simulink model "dspddc"  (Simulink 6.0)
settings: Solver=FixedStepDiscrete  SolverMode=SingleTasking  StartTime=0.0  StopTime=20500/69.333e6  RelTol=1e-3
PreLoadFcn:
  | gsmcoeffs
InitFcn:
  | ;fxptdlg('fxptdlg_simInit_cb');
StartFcn:
  | ;fxptdlg('fxptdlg_sim_cb');
StopFcn:
  | ;fxptdlg('fxptdlg_store_cb');
values from neighbouring files (symbols this model uses):
  cfir = [ -0.00073242187500  -0.00091552734375   0.00393676757813            0.01202392578125   0.00631713867188  -0.02673339843750           -0.05920410156250  -0.02371215820313   0.11474609375000            0.28945922851563   0.37011718750000   0.28945922851563            0.11474609375000  -0.02371215820313  -0.05920410156250           -0.02673339843750   0.00631713867188   0.01202392578125            0 ...(+54 chars)    [gsmcoeffs.m]
  pfir = [0.00073242187500   0.00213623046875  -0.00024414062500    -0.00253295898438  -0.00265502929688   0.00125122070313     0.00494384765625   0.00320434570313  -0.00338745117188     -0.00744628906250  -0.00314331054688   0.00601196289063    0.00991821289063   0.00292968750000  -0.00885009765625    -0.01293945312500  -0.00320434570313   0.01242065429688    0.01766967773438   0.00396728515625  -0.018188 ...(+835 chars)    [gsmcoeffs.m]
libraries: simulink x9, dspmlti3 x4, dspsigops x3, dspbuff3 x1, dspmlti4 x1, fixpt_lib_4 x1, dspsrcs4 x1, dspsnks4 x1, dspindex x1
PreSaveFcn:
  | ;fxptdlg('fxptdlg_presave_cb');
CloseFcn:
  | ;fxptdlg('fxptdlg_close_cb');
settings Model: MinMaxOverflowLogging=OverflowOnly  Creator=schim  LastModifiedBy=sconahan  ExtModeAutoUpdateStatusClock=off  ProdHWDeviceType=ASIC/FPGA
settings DataIOCC: LimitDataPoints=off  SaveOutput=off  SaveTime=off  SignalLoggingName=sigsOut
settings OptimizationCC: InlineParams=on
settings DebuggingCC: CheckExecutionContextPreStartOutputMsg=on  CheckExecutionContextRuntimeOutputMsg=on  SolverPrmCheckMsg=none  IntegerOverflowMsg=none  ParameterPrecisionLossMsg=none
settings HardwareCC: ProdHWDeviceType=ASIC/FPGA

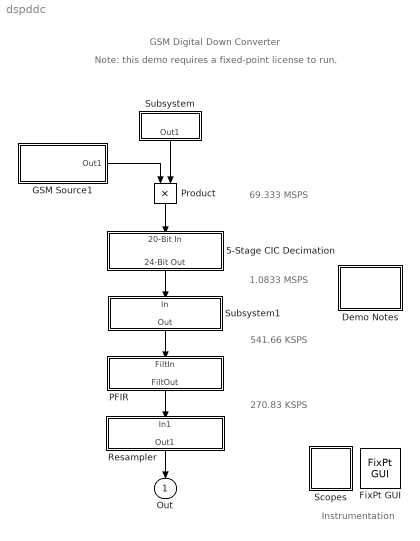
== system dspddc ==
  note: 1.0833
      | MSPS
  note: 541.66
      | KSPS
  note: 270.83
      | KSPS
  note: 69.333
      | MSPS
  note: Instrumentation
  note: GSM Digital Down Converter
  note: Note: this demo requires a fixed-point license to run.
  5-Stage CIC Decimation : Subsystem  Orientation=down  PropExecContextAcrossSSBoundary=on
      mask Display: disp('CIC Decimator')
  Demo Notes : Subsystem  PropExecContextAcrossSSBoundary=on
      settings: OpenFcn=web(which('dspddc.html'))
      mask Display: disp('Notes')
  FixPt GUI : fixpt_lib_4/FixPt GUI
  GSM Source1 : Subsystem  PropExecContextAcrossSSBoundary=on  mask(GSM Source){source_type=Chirp}
      mask prompts: source_type "Source type:"
      mask init:
      | pure_tune_input = (source_type - 1);
      mask StyleString: popup(Chirp|Sinusoid)
      mask Display:
      | disp(['GSM' 10 'Source']);
      | 
      | 
      | 
      | 
      | 
      | 
      | port_label('output', 1, 'A/D');
  PFIR : Subsystem  Orientation=down  PropExecContextAcrossSSBoundary=on  mask(PFIR){h=pfir, g=1024}
      mask prompts: h "PFIR coefficients:"; g "FINE gain (1-16383):"
      mask help: Valid FINE (gain parameter) inputs are positive integers less than 16383. The FINE_GAIN is calculated as FINE/1024.
      mask Display: disp('Programmable FIR')
  Product : Product  Orientation=down  OutDataTypeMode=Specify via dialog  OutDataType=sfix(20)  OutScaling=2^-18  RndMeth=Nearest
  Resampler : Subsystem  Orientation=down  PropExecContextAcrossSSBoundary=on  mask(Resampler){h=fir1(31,0.25), Ndelay=4, Ndec=3}
      mask prompts: h "Resampling FIR coefficients:"; Ndelay "NDELAY (upsample factor):"; Ndec "NDEC (downsample factor):"
      mask Display: disp('Rate Conversion')
  Scopes : Subsystem  PropExecContextAcrossSSBoundary=on
      mask Display: disp('Scopes')
  Subsystem : Subsystem  Orientation=down  PropExecContextAcrossSSBoundary=on  mask(Numerically Controlled Oscillator (NCO)){tune_freq=(5/24) * (2^32), phase_offset=0, enable_dither=on, bits=5}
      mask prompts: tune_freq "Normalized 32-bit tuning frequency (0 to 2^32)"; phase_offset "Normalized 16-bit phase offset (0 to 2^16):"; enable_dither "Enable dithering"; bits "Number of dither bits (1 to 19):"
      mask Display: disp('NCO')
  Subsystem1 : Subsystem  Orientation=down  PropExecContextAcrossSSBoundary=on  mask(Compensation FIR (CFIR)){coarse_gain=0, cfir_h=cfir}
      mask prompts: coarse_gain "COARSE gain (0-7):"; cfir_h "CFIR coefficients:"
      mask Display: disp('Compensation FIR')
  Out : Outport  Orientation=down
  wires:
  Product/1 -> 5-Stage CIC Decimation/1(20-Bit In)
  Subsystem/1(Out1) -> Product/2
  GSM Source1/1(Out1) -> Product/1
  Subsystem1/1(Out) -> PFIR/1(FiltIn)
  PFIR/1(FiltOut) -> Resampler/1(In1)
  Resampler/1(Out1) -> Out/1
  5-Stage CIC Decimation/1(24-Bit Out) -> Subsystem1/1(In)

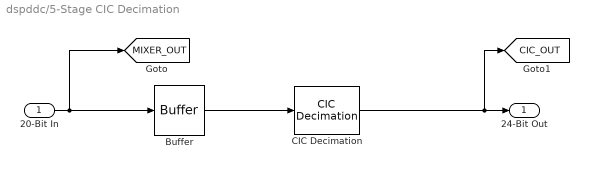
== system dspddc/5-Stage CIC Decimation ==
  20-Bit In : Inport  LatchInput=off
  Buffer : dspbuff3/Buffer  N=64  V=0  ic=0
  CIC Decimation : dspmlti4/CIC Decimation  filtFrom=Dialog  filtobj=Hm_decim  ftype=Decimator  R=64  resampPhase=0  M=1  N=5  BPS=[50 29 24 24 24 24 24 24 24 24]  launchFVT=off  framing=Maintain input frame rate
  24-Bit Out : Outport
  tag scope: CIC_OUT=global, MIXER_OUT=global
  wires:
  20-Bit In/1 -> [MIXER_OUT], Buffer/1
  Buffer/1 -> CIC Decimation/1
  CIC Decimation/1 -> 24-Bit Out/1, [CIC_OUT]

== system dspddc/Demo Notes ==

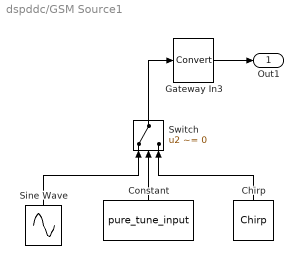
== system dspddc/GSM Source1 ==
  Chirp : dspsrcs4/Chirp  Orientation=up  sweep=Linear  mode=Unidirectional  f0=.2078*69.333e6  f1=.2088*69.333e6  t1=16384/69.333e6  Tsweep=16384/69.333e6  phase=0  Ts=1/69.333e6  spf=1  datatype=Double
  Constant : Constant  Orientation=up  Value=pure_tune_input  OutDataTypeMode=boolean
  Gateway In3 : DataTypeConversion  OutDataTypeMode=Specify via dialog  OutDataType=sfix(14)  OutScaling=2^-13  RndMeth=Nearest  SaturateOnIntegerOverflow=on
  Sine Wave : Sin  Orientation=up  Frequency=2*pi*69.1e6*5/24  SampleTime=1/69.333e6
  Switch : Switch  Orientation=up  Criteria=u2 ~= 0  Threshold=0.5  InputSameDT=on
  Out1 : Outport
  wires:
  Switch/1 -> Gateway In3/1
  Sine Wave/1 -> Switch/1
  Chirp/1 -> Switch/3
  Constant/1 -> Switch/2
  Gateway In3/1 -> Out1/1

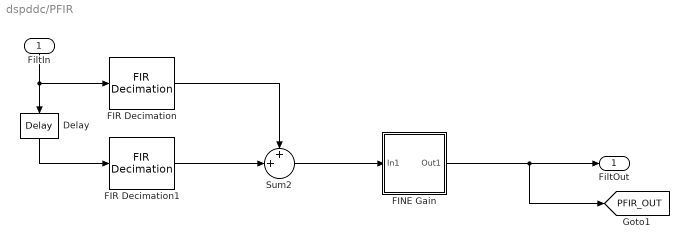
== system dspddc/PFIR ==
  FiltIn : Inport  Orientation=down  LatchInput=off
  Delay : dspsigops/Delay  Orientation=down  dly_unit=Samples  delay=1  ic_detail=off  dif_ic_for_ch=off  dif_ic_for_dly=off  ic=0  reset_popup=None
  FINE Gain : Subsystem  PropExecContextAcrossSSBoundary=on
      mask Display: disp('FINE\nGain')
  FIR Decimation : dspmlti3/FIR Decimation  DialogController=dspDDGCreate  DialogControllerArgs=DataTag1  h=h(1:2:length(h))  D=2  framing=Maintain input frame size  outputBufInitCond=0  firstCoeffMode=Specify word length  firstCoeffWordLength=16  firstCoeffFracLength=16  prodOutputMode=Binary point scaling  prodOutputWordLength=20  prodOutputFracLength=-12  roundingMode=Nearest  overflowMode=off
  FIR Decimation1 : dspmlti3/FIR Decimation  DialogController=dspDDGCreate  DialogControllerArgs=DataTag2  h=h(2:2:length(h))  D=2  framing=Maintain input frame size  outputBufInitCond=0  firstCoeffMode=Specify word length  firstCoeffWordLength=16  firstCoeffFracLength=16  prodOutputMode=Binary point scaling  prodOutputWordLength=20  prodOutputFracLength=-12  roundingMode=Nearest  overflowMode=off
  Sum2 : Sum  Inputs=++|  OutDataType=sfix(20)  OutScaling=2^12  SaturateOnIntegerOverflow=on  InputSameDT=on
  FiltOut : Outport
  tag scope: PFIR_OUT=global
  wires:
  Delay/1 -> FIR Decimation1/1
  FIR Decimation/1 -> Sum2/1
  FIR Decimation1/1 -> Sum2/2
  FiltIn/1 -> Delay/1, FIR Decimation/1
  Sum2/1 -> FINE Gain/1(In1)
  FINE Gain/1(Out1) -> FiltOut/1, [PFIR_OUT]

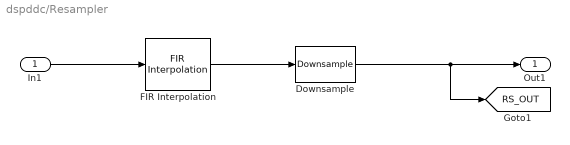
== system dspddc/Resampler ==
  In1 : Inport  LatchInput=off
  Downsample : dspsigops/Downsample  N=Ndec  phase=0  ic=0  smode=Allow multirate  fmode=Maintain input frame size
  FIR Interpolation : dspmlti3/FIR Interpolation  DialogController=dspDDGCreate  DialogControllerArgs=DataTag3  h=h  L=Ndelay  framing=Maintain input frame size  outputBufInitCond=0  firstCoeffMode=Specify word length  firstCoeffWordLength=12  firstCoeffFracLength=13  prodOutputMode=Binary point scaling  prodOutputWordLength=24  prodOutputFracLength=-12  roundingMode=Nearest  overflowMode=off
  Out1 : Outport
  tag scope: RS_OUT=global
  wires:
  In1/1 -> FIR Interpolation/1
  Downsample/1 -> [RS_OUT], Out1/1
  FIR Interpolation/1 -> Downsample/1

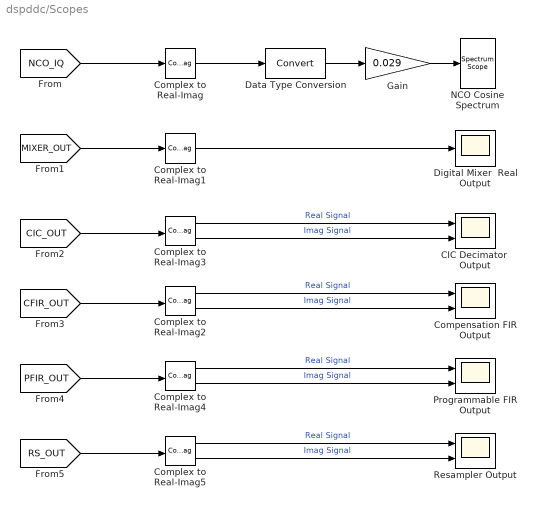
== system dspddc/Scopes ==
  CIC Decimator  Output : Scope  NumInputPorts=2
      settings: TimeRange=0.0003  YMin=-1e+009~-1e+009  YMax=1e+009~1e+009  DataFormat=Structure  MaxDataPoints=1000000
  Compensation FIR Output : Scope  NumInputPorts=2
      settings: TimeRange=0.0003  YMin=-1e+009~-1e+009  YMax=1e+009~1e+009  SaveName=ScopeData2  DataFormat=Structure  MaxDataPoints=1000000
  Complex to Real-Imag : ComplexToRealImag  Output=Real
  Complex to Real-Imag1 : ComplexToRealImag  Output=Real
  Complex to Real-Imag{2..5} (4 alike) : ComplexToRealImag
  Data Type Conversion : DataTypeConversion  OutDataTypeMode=double  SaturateOnIntegerOverflow=on  RndMeth=Zero
  Digital Mixer  Real Output : Scope
      settings: TimeRange=0.0003  YMin=-1  YMax=1  SaveName=ScopeData5  DataFormat=Structure  MaxDataPoints=1000000
  Gain : Gain  Gain=0.029  SaturateOnIntegerOverflow=on
  NCO Cosine Spectrum : dspsnks4/Spectrum Scope  ScopeProperties=on  Domain=Frequency  HorizSpan=1  UseBuffer=on  BufferSize=8192  Overlap=0  inpFftLenInherit=off  FFTlength=128  numAvg=2  DisplayProperties=off  AxisGrid=on  Memory=off  FrameNumber=off  AxisLegend=off  AxisZoom=off  OpenScopeAtSimStart=on  OpenScopeImmediately=off  FigPos=[19 48 560 420]  AxisProperties=off  XUnits=Hertz  XRange=[0...Fs/2]  InheritXIncr=on  XIncr=1.0  XLabel=Samples  YUnits=dB  YLabel=Magnitude, dB  LineProperties=off
      settings: YMin=-160  YMax=5
  Programmable FIR Output : Scope  NumInputPorts=2
      settings: TimeRange=0.0003  YMin=-1e+009~-1e+009  YMax=1e+009~1e+009  SaveName=ScopeData3  DataFormat=Structure  MaxDataPoints=1000000
  Resampler Output : Scope  NumInputPorts=2
      settings: TimeRange=0.0003  YMin=-2e+008~-2e+008  YMax=2e+008~2e+008  SaveName=ScopeData4  DataFormat=Structure  MaxDataPoints=1000000
  wires:
  Complex to Real-Imag/1 -> Data Type Conversion/1
  Gain/1 -> NCO Cosine Spectrum/1
  [NCO_IQ] -> Complex to Real-Imag/1
  Data Type Conversion/1 -> Gain/1
  [MIXER_OUT] -> Complex to Real-Imag1/1
  Complex to Real-Imag1/1 -> Digital Mixer  Real Output/1
  Complex to Real-Imag3/1 -> CIC Decimator  Output/1  "Real Signal"
  Complex to Real-Imag3/2 -> CIC Decimator  Output/2  "Imag Signal"
  [CIC_OUT] -> Complex to Real-Imag3/1
  Complex to Real-Imag2/1 -> Compensation FIR Output/1  "Real Signal"
  Complex to Real-Imag2/2 -> Compensation FIR Output/2  "Imag Signal"
  [CFIR_OUT] -> Complex to Real-Imag2/1
  Complex to Real-Imag4/1 -> Programmable FIR Output/1  "Real Signal"
  Complex to Real-Imag4/2 -> Programmable FIR Output/2  "Imag Signal"
  [PFIR_OUT] -> Complex to Real-Imag4/1
  Complex to Real-Imag5/1 -> Resampler Output/1  "Real Signal"
  Complex to Real-Imag5/2 -> Resampler Output/2  "Imag Signal"
  [RS_OUT] -> Complex to Real-Imag5/1

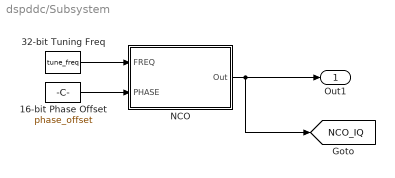
== system dspddc/Subsystem ==
  16-bit Phase Offset : Constant  Value=phase_offset  OutDataTypeMode=Specify via dialog  OutDataType=ufix(16)  OutScaling=2^-0
  32-bit Tuning Freq : Constant  Value=tune_freq  OutDataTypeMode=Specify via dialog  OutDataType=ufix(32)  OutScaling=2^-0
  NCO : Subsystem  PropExecContextAcrossSSBoundary=on
      mask Type: Numerically Controlled Oscillator (NCO)
      mask Display: disp('NCO')
  Out1 : Outport
  tag scope: NCO_IQ=global
  wires:
  16-bit Phase Offset/1 -> NCO/2(PHASE)
  32-bit Tuning Freq/1 -> NCO/1(FREQ)
  NCO/1(Out) -> Out1/1, [NCO_IQ]

== system dspddc/Subsystem1 ==
  In : Inport  LatchInput=off
  Coarse Gain : Subsystem  PropExecContextAcrossSSBoundary=on
      mask Display: disp(['Coarse' 10 'Gain'])
  FIR Decimation : dspmlti3/FIR Decimation  DialogController=dspDDGCreate  DialogControllerArgs=DataTag4  h=cfir_h  D=2  framing=Maintain input frame size  outputBufInitCond=0  firstCoeffMode=Specify word length  firstCoeffWordLength=16  firstCoeffFracLength=16  prodOutputMode=Binary point scaling  prodOutputWordLength=20  prodOutputFracLength=-12  roundingMode=Nearest  overflowMode=off
  Out : Outport
  tag scope: CFIR_OUT=global
  wires:
  Coarse Gain/1(20-Bit Out) -> FIR Decimation/1
  In/1 -> Coarse Gain/1(24-Bit In)
  FIR Decimation/1 -> Out/1, [CFIR_OUT]

== system dspddc/PFIR/FINE Gain ==
  In1 : Inport  LatchInput=off
  Conversion : DataTypeConversion  OutDataTypeMode=Specify via dialog  OutDataType=sfix(24)  OutScaling=2^12
  Shift Arithmetic : simulink/Logic and Bit Operations/Shift Arithmetic  nBitShiftRight=-( log2(g) - 10 )  nBinPtShiftRight=0
  Out1 : Outport
  wires:
  Conversion/1 -> Shift Arithmetic/1
  In1/1 -> Conversion/1
  Shift Arithmetic/1 -> Out1/1

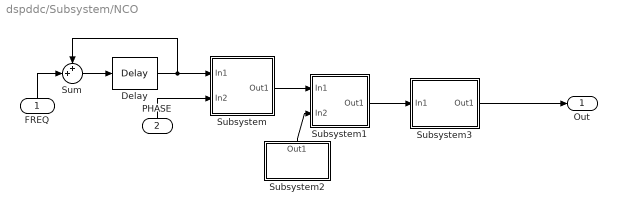
== system dspddc/Subsystem/NCO ==
  FREQ : Inport  Orientation=up  LatchInput=off
  PHASE : Inport  Orientation=up  Port=2  LatchInput=off
  Delay : dspsigops/Delay  dly_unit=Samples  delay=1  ic_detail=off  dif_ic_for_ch=off  dif_ic_for_dly=off  ic=0  reset_popup=None
  Subsystem : Subsystem  PropExecContextAcrossSSBoundary=on
      mask Display: disp(['Sum and\nretain\n23 MSBs'])
  Subsystem1 : Subsystem  PropExecContextAcrossSSBoundary=on
      mask Display: disp('Sum and\nretain\n18 MSBs')
  Subsystem2 : Subsystem  Orientation=up  PropExecContextAcrossSSBoundary=on
      mask Display: disp(['Dither' 10 'Generator'])
  Subsystem3 : Subsystem  PropExecContextAcrossSSBoundary=on
      mask Display: disp(['Sine/Cosine\nLookup'])
  Sum : Sum  Inputs=++|  OutDataTypeMode=uint32  RndMeth=Nearest
  Out : Outport
  wires:
  FREQ/1 -> Sum/2
  Delay/1 -> Subsystem/1(In1), Sum/1
  PHASE/1 -> Subsystem/2(In2)
  Sum/1 -> Delay/1
  Subsystem/1(Out1) -> Subsystem1/1(In1)
  Subsystem1/1(Out1) -> Subsystem3/1(In1)
  Subsystem2/1(Out1) -> Subsystem1/2(In2)
  Subsystem3/1(Out1) -> Out/1

== system dspddc/Subsystem1/Coarse Gain ==
  24-Bit In : Inport  LatchInput=off
  Conversion : DataTypeConversion  OutDataTypeMode=Specify via dialog  OutDataType=sfix(24)  OutScaling=2^12
  Extract Bits : simulink/Logic and Bit Operations/Extract Bits  bitsToExtract=Range of bits  numBits=8  bitIdxRange=[0 19]  outScalingMode=Preserve fixed-point scaling
  Shift Arithmetic : simulink/Logic and Bit Operations/Shift Arithmetic  nBitShiftRight=-1*coarse_gain  nBinPtShiftRight=0
  20-Bit Out : Outport
  wires:
  Shift Arithmetic/1 -> Conversion/1
  24-Bit In/1 -> Shift Arithmetic/1
  Extract Bits/1 -> 20-Bit Out/1
  Conversion/1 -> Extract Bits/1

== system dspddc/Subsystem/NCO/Subsystem ==
  In1 : Inport  LatchInput=off
  In2 : Inport  Port=2  LatchInput=off
  Add : Sum  Inputs=|++  OutDataTypeMode=Specify via dialog  OutDataType=ufix(32)  OutScaling=2^-0
  Retain 23 MSBs : Subsystem  PropExecContextAcrossSSBoundary=on
  Out1 : Outport
  wires:
  Add/1 -> Retain 23 MSBs/1(In)
  In1/1 -> Add/1
  Retain 23 MSBs/1(Out) -> Out1/1
  In2/1 -> Add/2

== system dspddc/Subsystem/NCO/Subsystem1 ==
  In1 : Inport  LatchInput=off
  In2 : Inport  Port=2  LatchInput=off
  Add1 : Sum  Inputs=|++  OutDataTypeMode=Specify via dialog  OutDataType=ufix(23)  OutScaling=2^-0  InputSameDT=on
  Retain 18 MSBs : Subsystem  PropExecContextAcrossSSBoundary=on
  Out1 : Outport
  wires:
  Add1/1 -> Retain 18 MSBs/1(In)
  Retain 18 MSBs/1(Out) -> Out1/1
  In1/1 -> Add1/1
  In2/1 -> Add1/2

== system dspddc/Subsystem/NCO/Subsystem2 ==
  Constant : Constant  Orientation=up  Value=enable_dither  OutDataTypeMode=boolean
  Constant1 : Constant  Orientation=up  Value=0  OutDataTypeMode=Specify via dialog  OutDataType=ufix(23)
  Dither1 : Subsystem  Orientation=up  PropExecContextAcrossSSBoundary=on
      mask Display: disp(['DITHER' 10 'GENERATOR'])
  Switch : Switch  Orientation=up  Criteria=u2 ~= 0  Threshold=0.5  InputSameDT=on
  Out1 : Outport  Orientation=up
  wires:
  Constant/1 -> Switch/2
  Constant1/1 -> Switch/3
  Dither1/1(Out1) -> Switch/1
  Switch/1 -> Out1/1

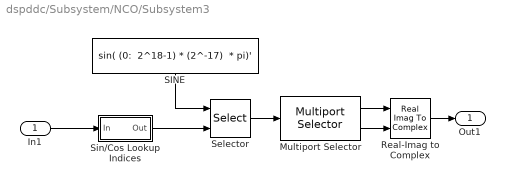
== system dspddc/Subsystem/NCO/Subsystem3 ==
  In1 : Inport  LatchInput=off
  Multiport Selector : dspindex/Multiport Selector  rowsOrCols=Rows  idxCellArray={ 1, 2 }  idxErrMode=Clip Index
  Real-Imag to Complex : RealImagToComplex
  SINE : Constant  Orientation=down  Value="sin( (0:  2^18-1) * (2^-17)  * pi)'"  VectorParams1D=off  OutDataTypeMode=Specify via dialog  OutDataType=sfix(20)  OutScaling=2^-18
  Selector : Selector  ElementSrc=External  Elements=[1 3]  InputPortWidth=2^18
  Sin/Cos Lookup Indices : Subsystem  PropExecContextAcrossSSBoundary=on
  Out1 : Outport
  wires:
  SINE/1 -> Selector/1
  Sin/Cos Lookup Indices/1(Out) -> Selector/2
  In1/1 -> Sin/Cos Lookup Indices/1(In)
  Selector/1 -> Multiport Selector/1
  Multiport Selector/1 -> Real-Imag to Complex/1
  Multiport Selector/2 -> Real-Imag to Complex/2
  Real-Imag to Complex/1 -> Out1/1

== system dspddc/Subsystem/NCO/Subsystem/Retain 23 MSBs ==
  In : Inport  LatchInput=off
  Conversion : DataTypeConversion  OutDataTypeMode=Specify via dialog  OutDataType=ufix(23)  OutScaling=2^9
  Conversion1 : DataTypeConversion  OutDataTypeMode=Specify via dialog  OutDataType=ufix(23)  ConvertRealWorld=Stored Integer (SI)
  Out : Outport
  wires:
  Conversion/1 -> Conversion1/1
  Conversion1/1 -> Out/1
  In/1 -> Conversion/1

== system dspddc/Subsystem/NCO/Subsystem1/Retain 18 MSBs ==
  In : Inport  LatchInput=off
  Conversion : DataTypeConversion  OutDataTypeMode=Specify via dialog  OutDataType=ufix(23)  OutScaling=2^5
  Conversion1 : DataTypeConversion  OutDataTypeMode=Specify via dialog  OutDataType=ufix(18)  ConvertRealWorld=Stored Integer (SI)
  Out : Outport
  wires:
  Conversion/1 -> Conversion1/1
  Conversion1/1 -> Out/1
  In/1 -> Conversion/1

== system dspddc/Subsystem/NCO/Subsystem2/Dither1 ==
  Gateway In3 : DataTypeConversion  OutDataTypeMode=Specify via dialog  OutDataType=ufix(23)
  Shift Arithmetic : simulink/Logic and Bit Operations/Shift Arithmetic  nBitShiftRight=(19-bits)  nBinPtShiftRight=0
  Subsystem : Subsystem  PropExecContextAcrossSSBoundary=on  mask{nbit=19, ts=1/69.333e6}
      mask prompts: nbit "Shift register size (nbits):"; ts "Sample time:"
      mask Display: disp(['Fixed-point' 10 'Random' 10 'Number' 10 'Generator'])
  Out1 : Outport
  wires:
  Gateway In3/1 -> Out1/1
  Subsystem/1(Out1) -> Shift Arithmetic/1
  Shift Arithmetic/1 -> Gateway In3/1

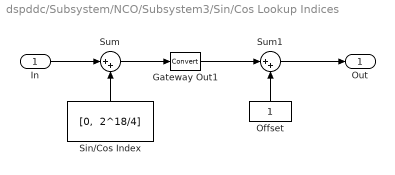
== system dspddc/Subsystem/NCO/Subsystem3/Sin/Cos Lookup Indices ==
  In : Inport  LatchInput=off
  Gateway Out1 : DataTypeConversion  OutDataTypeMode=uint32  ConvertRealWorld=Stored Integer (SI)
  Offset : Constant  Orientation=up  OutDataTypeMode=Specify via dialog  OutDataType=uint(32)  OutScaling=2^-0
  Sin/Cos Index : Constant  Orientation=up  Value="[0,  2^18/4]"  OutDataType=sfix(5)  OutScaling=2^-0
  Sum : Sum  Inputs=|++  InputSameDT=on
  Sum1 : Sum  Inputs=|++  InputSameDT=on
  Out : Outport
  wires:
  Sum/1 -> Gateway Out1/1
  In/1 -> Sum/1
  Sin/Cos Index/1 -> Sum/2
  Sum1/1 -> Out/1
  Gateway Out1/1 -> Sum1/1
  Offset/1 -> Sum1/2

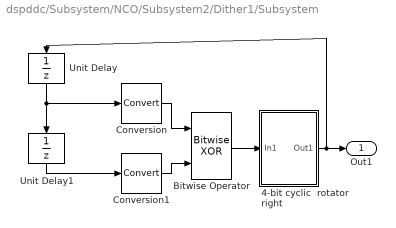
== system dspddc/Subsystem/NCO/Subsystem2/Dither1/Subsystem ==
  4-bit cyclic  rotator right : Subsystem  PropExecContextAcrossSSBoundary=on
      mask Display: disp(['Cyclic' 10 'Right' 10 'Rotator' 10 'ROR'])
  Bitwise Operator : simulink/Logic and Bit Operations/Bitwise Operator  logicop=XOR  UseBitMask=off  NumInputPorts=2  BitMask=bin2dec('11011001')  BitMaskRealWorld=Stored Integer
  Conversion : DataTypeConversion  OutDataTypeMode=Specify via dialog  OutDataType=ufix(nbit)
  Conversion1 : DataTypeConversion  OutDataTypeMode=Specify via dialog  OutDataType=ufix(nbit)
  Unit Delay : UnitDelay  Orientation=down  X0=1  SampleTime=ts
  Unit Delay1 : UnitDelay  Orientation=down  X0=2  SampleTime=ts
  Out1 : Outport
  wires:
  Unit Delay1/1 -> Conversion1/1
  Conversion1/1 -> Bitwise Operator/2
  Conversion/1 -> Bitwise Operator/1
  4-bit cyclic  rotator right/1(Out1) -> Unit Delay/1, Out1/1
  Bitwise Operator/1 -> 4-bit cyclic  rotator right/1(In1)
  Unit Delay/1 -> Conversion/1, Unit Delay1/1

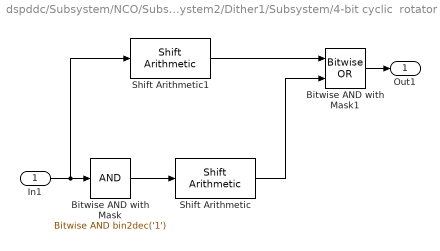
== system dspddc/Subsystem/NCO/Subsystem2/Dither1/Subsystem/4-bit cyclic  rotator right ==
  In1 : Inport  LatchInput=off
  Bitwise AND with Mask : simulink/Logic and Bit Operations/Bitwise Operator  logicop=AND  UseBitMask=on  BitMask=bin2dec('1')  BitMaskRealWorld=Stored Integer
  Bitwise AND with Mask1 : simulink/Logic and Bit Operations/Bitwise Operator  logicop=OR  UseBitMask=off  NumInputPorts=2  BitMask=bin2dec('1')  BitMaskRealWorld=Stored Integer
  Shift Arithmetic : simulink/Logic and Bit Operations/Shift Arithmetic  nBitShiftRight=-(nbit-1)  nBinPtShiftRight=0
  Shift Arithmetic1 : simulink/Logic and Bit Operations/Shift Arithmetic  nBitShiftRight=1  nBinPtShiftRight=0
  Out1 : Outport
  wires:
  In1/1 -> Shift Arithmetic1/1, Bitwise AND with Mask/1
  Bitwise AND with Mask/1 -> Shift Arithmetic/1
  Shift Arithmetic/1 -> Bitwise AND with Mask1/2
  Shift Arithmetic1/1 -> Bitwise AND with Mask1/1
  Bitwise AND with Mask1/1 -> Out1/1
